simulink model "SimpleEKF_2007a"  (Simulink 6.6)
settings: Solver=FixedStepDiscrete  StartTime=0.0  StopTime=300  FixedStep=0.01  RelTol=1e-3
values from neighbouring files (symbols this model uses):
  initP = diag([ 1 1 1 1e5 1e5 1 1e5 1e5 1e5 ])    [SimpleEKF_init.m.m]
undefined symbols (not defined in the file or in its folder): DiscIntNeverNeededParam, gcbh, hwbcalib_subsystem
libraries: simulink x8, dspmtrx3 x5, dspinverses x1
(part 4 of 9)

== system SimpleEKF_2007a/INS/Coriolis correction/skewSymmetric1 ==
  skewLibIn : Inport  OutDataType=fixdt(1,16,0)  OutScaling=[]
  column1 : Selector  Tag=MBDLibrary v2007b.1  IndexOptions=Index vector (dialog)  Indices=[7 3 5]  OutputSizes=1  InputPortWidth=7  mask(Mux Selector (MBDLibrary)){InputPortWidth_mbdlib=7, Indices_mbdlib=[7 3 5]}
      mask prompts: InputPortWidth_mbdlib "Input Port Width"; Indices_mbdlib "Output Indices"
      mask help: Changes the order of the inputs.
      settings: OpenFcn=|
      | if exist('mbdlib_dialog')
      |    mbdlib_dialog(gcb,'open')
      | else
      |    open_system(gcb, 'mask')
      | end
      settings: CloseFcn=|
      | if exist('mbdlib_selector')
      |    mbdlib_selector(gcb)
      | end
      mask Help: The SELECTOR block is a MULTIPLEXED SELECTOR block, used to change the input/output order of a multiplexed data stream.
      mask Display:
      | port_label('input', 1,'[7]')
      | text(1.0,0.83333,'7', 'horizontalAlignment', 'right')
      | text(1.0,0.5,'3', 'horizontalAlignment', 'right')
      | text(1.0,0.16667,'5', 'horizontalAlignment', 'right')
  column2 : Selector  Tag=MBDLibrary v2007b.1  IndexOptions=Index vector (dialog)  Indices=[6 7 1]  OutputSizes=1  InputPortWidth=7  mask(Mux Selector (MBDLibrary)){InputPortWidth_mbdlib=7, Indices_mbdlib=[6 7 1]}
      mask prompts: InputPortWidth_mbdlib "Input Port Width"; Indices_mbdlib "Output Indices"
      mask help: Changes the order of the inputs.
      settings: OpenFcn=|
      | if exist('mbdlib_dialog')
      |    mbdlib_dialog(gcb,'open')
      | else
      |    open_system(gcb, 'mask')
      | end
      settings: CloseFcn=|
      | if exist('mbdlib_selector')
      |    mbdlib_selector(gcb)
      | end
      mask Help: The SELECTOR block is a MULTIPLEXED SELECTOR block, used to change the input/output order of a multiplexed data stream.
      mask Display:
      | port_label('input', 1,'[7]')
      | text(1.0,0.83333,'6', 'horizontalAlignment', 'right')
      | text(1.0,0.5,'7', 'horizontalAlignment', 'right')
      | text(1.0,0.16667,'1', 'horizontalAlignment', 'right')
  column3 : Selector  Tag=MBDLibrary v2007b.1  IndexOptions=Index vector (dialog)  Indices=[2 4 7]  OutputSizes=1  InputPortWidth=7  mask(Mux Selector (MBDLibrary)){InputPortWidth_mbdlib=7, Indices_mbdlib=[2 4 7]}
      mask prompts: InputPortWidth_mbdlib "Input Port Width"; Indices_mbdlib "Output Indices"
      mask help: Changes the order of the inputs.
      settings: OpenFcn=|
      | if exist('mbdlib_dialog')
      |    mbdlib_dialog(gcb,'open')
      | else
      |    open_system(gcb, 'mask')
      | end
      settings: CloseFcn=|
      | if exist('mbdlib_selector')
      |    mbdlib_selector(gcb)
      | end
      mask Help: The SELECTOR block is a MULTIPLEXED SELECTOR block, used to change the input/output order of a multiplexed data stream.
      mask Display:
      | port_label('input', 1,'[7]')
      | text(1.0,0.83333,'2', 'horizontalAlignment', 'right')
      | text(1.0,0.5,'4', 'horizontalAlignment', 'right')
      | text(1.0,0.16667,'7', 'horizontalAlignment', 'right')
  matrixConcat : Concatenate  Tag=MBDLibrary v2007b.1  NumInputs=3  Mode=Multidimensional array  ConcatenateDimension=2  mask(Matrix Concat (MBDLibrary)){concatDim=Horizontal, numInputs_mbdlib=3}
      mask prompts: concatDim "Type of Concatenate"; numInputs_mbdlib "Number of Inputs"
      mask help: Concatenate input signals of the same data type to create a contiguous output signal.
      settings: OpenFcn=|
      | if exist('mbdlib_dialog')
      |    mbdlib_dialog(gcb,'open')
      | else
      |    open_system(gcb, 'mask')
      | end
      settings: CloseFcn=|
      | if exist('mbdlib_matrixConcatenate')
      |    mbdlib_matrixConcatenate(gcb, 'mask')
      | end
      mask Help:
      | The MATRIX CONCAT block concatenates input signals from the dame data type and creates a contigouos output matrix.
      | In vector mode, all input signals must be either vectors or one-row [1xM] matrices or one-column [Mx1] matrices or a combination of vectors and either one-row matrices or one-column matrices. The output is a vector if all inputs are vectors. The output is a one-row or one-column matrix if any of the inputs are one-row or one-column matrices respectively.
      | 
      | Matrix mode treats vector inputs as one-column matrices. The output is always a matrix.
      mask StyleString: popup(Vertical|Horizontal),edit
      mask Display:
      | plot([0.1 0.3 0.3 0.1 0.1], [0.1 0.1 0.9 0.9 0.1])
      | plot([0.4 0.6 0.6 0.4 0.4], [0.1 0.1 0.9 0.9 0.1])
      | plot([0.7 0.9 0.9 0.7 0.7], [0.1 0.1 0.9 0.9 0.1])
  mux : Mux  Tag=MBDLibrary v2007b.1  Inputs=3  mask(Mux (MBDLibrary)){Inputs_mbdlib=3}
      mask prompts: Inputs_mbdlib "Number of Inputs"
      mask help: Converts multipule inputs to a vector.
      settings: OpenFcn=|
      | if exist('mbdlib_dialog')
      |    mbdlib_dialog(gcb,'open')
      | else
      |    open_system(gcb, 'mask')
      | end
      mask Help: The MUX block provides a vector output to the model for separate inputs.  The output order will correspond to the input order (from the first input at the top of the block to the last input at the bottom of the block).
  negative : Gain  Tag=MBDLibrary v2007b.1  Gain=-1  ParameterDataType=fixdt(1,16,0)  ParameterScaling=[]  OutDataType=fixdt(1,16,0)  OutScaling=[]  RndMeth=Zero  mask(Gain (MBDLibrary)){gain_mbdlib=-1}
      mask prompts: gain_mbdlib "Gain"
      mask help: Multiplies the input by the gain.
      settings: OpenFcn=|
      | if exist('mbdlib_dialog')
      |    mbdlib_dialog(gcb,'open')
      | else
      |    open_system(gcb, 'mask')
      | end
      mask Help: The GAIN block multiplies the input by the gain value.  This block may accept any data types other than boolean.  The user must take care to not use a non-integer gain for int32/uint32 inputs.
      mask Display: disp([get_param(gcb, 'Gain') 'x'])
  zero : Constant  Tag=MBDLibrary v2007b.1  Value=0  VectorParams1D=off  OutDataType=fixdt(1,16,0)  OutScaling=[]  mask(Constant (MBDLibrary)){Value_mbdlib=0, OutDataTypeMode_mbdlib=double}
      mask prompts: Value_mbdlib "Constant"; OutDataTypeMode_mbdlib "Data Type"
      mask help: Outputs a constant value
      settings: AttributesFormatString={%<OutDataTypeMode>}
      settings: OpenFcn=|
      | if exist('mbdlib_dialog')
      |    mbdlib_dialog(gcb,'open')
      | else
      |    open_system(gcb, 'mask')
      | end
      settings: CloseFcn=|
      | if exist('mbdlib_dialog')
      |    mbdlib_constant(gcb)
      | end
      mask Help: The CONSTANT block outputs a constant value to the system.
      mask StyleString: edit,popup(double|single|boolean|int32|uint32)
  skewLibOut : Outport  OutDataType=fixdt(1,16,0)  OutScaling=[]
  wires:
  zero/1 -> mux/3
  negative/1 -> mux/2
  column3/1 -> matrixConcat/3
  column2/1 -> matrixConcat/2
  column1/1 -> matrixConcat/1
  matrixConcat/1 -> skewLibOut/1
  mux/1 -> column1/1, column3/1, column2/1
  skewLibIn/1 -> mux/1, negative/1

== system SimpleEKF_2007a/INS/Gravity/square ==
  squareLibIn : Inport  DataType=double  OutDataType=fixdt(1,16,0)  OutScaling=[]
  Product : Product  OutDataType=fixdt(1,16,0)  OutScaling=[]  RndMeth=Zero
  squareLibOut : Outport  OutDataType=fixdt(1,16,0)  OutScaling=[]  InitialOutput=0
  wires:
  squareLibIn/1 -> Product/2, Product/1
  Product/1 -> squareLibOut/1

== system SimpleEKF_2007a/INS/Gravity/square1 ==
  squareLibIn : Inport  DataType=double  OutDataType=fixdt(1,16,0)  OutScaling=[]
  Product : Product  OutDataType=fixdt(1,16,0)  OutScaling=[]  RndMeth=Zero
  squareLibOut : Outport  OutDataType=fixdt(1,16,0)  OutScaling=[]  InitialOutput=0
  wires:
  squareLibIn/1 -> Product/2, Product/1
  Product/1 -> squareLibOut/1

== system SimpleEKF_2007a/INS/Gravity/square2 ==
  squareLibIn : Inport  DataType=double  OutDataType=fixdt(1,16,0)  OutScaling=[]
  Product : Product  OutDataType=fixdt(1,16,0)  OutScaling=[]  RndMeth=Zero
  squareLibOut : Outport  OutDataType=fixdt(1,16,0)  OutScaling=[]  InitialOutput=0
  wires:
  squareLibIn/1 -> Product/2, Product/1
  Product/1 -> squareLibOut/1

== system SimpleEKF_2007a/INS/Gravity/square3 ==
  squareLibIn : Inport  DataType=double  OutDataType=fixdt(1,16,0)  OutScaling=[]
  Product : Product  OutDataType=fixdt(1,16,0)  OutScaling=[]  RndMeth=Zero
  squareLibOut : Outport  OutDataType=fixdt(1,16,0)  OutScaling=[]  InitialOutput=0
  wires:
  squareLibIn/1 -> Product/2, Product/1
  Product/1 -> squareLibOut/1

== system SimpleEKF_2007a/INS/Gravity/square4 ==
  squareLibIn : Inport  DataType=double  OutDataType=fixdt(1,16,0)  OutScaling=[]
  Product : Product  OutDataType=fixdt(1,16,0)  OutScaling=[]  RndMeth=Zero
  squareLibOut : Outport  OutDataType=fixdt(1,16,0)  OutScaling=[]  InitialOutput=0
  wires:
  squareLibIn/1 -> Product/2, Product/1
  Product/1 -> squareLibOut/1

== system SimpleEKF_2007a/INS/Velocity update/acc from BODY to NAV ==
  acc_Body : Inport  PortDimensions=3  SampleTime=0.01  OutDataType=fixdt(1,16,0)  OutScaling=[]
  dcmBodyToNav : Inport  Port=2  PortDimensions=[3,3]  SampleTime=0.01  OutDataType=fixdt(1,16,0)  OutScaling=[]
  Matrix Multiply : Product  Multiplication=Matrix(*)  OutDataType=fixdt(1,16,0)  OutScaling=[]
  acc_Nav : Outport  PortDimensions=3  SampleTime=0.01  OutDataType=fixdt(1,16,0)  OutScaling=[]
  wires:
  dcmBodyToNav/1 -> Matrix Multiply/1
  Matrix Multiply/1 -> acc_Nav/1
  acc_Body/1 -> Matrix Multiply/2

== system SimpleEKF_2007a/INS/Velocity update/acc(k-1) from BODY to NAV ==
  acc_Body : Inport  OutDataType=fixdt(1,16,0)  OutScaling=[]
  dcmBodyToNav : Inport  Port=2  OutDataType=fixdt(1,16,0)  OutScaling=[]
  Matrix Multiply : Product  Multiplication=Matrix(*)  OutDataType=fixdt(1,16,0)  OutScaling=[]
  acc_Nav(k-1) : Outport  OutDataType=fixdt(1,16,0)  OutScaling=[]
  wires:
  dcmBodyToNav/1 -> Matrix Multiply/1
  Matrix Multiply/1 -> acc_Nav(k-1)/1
  acc_Body/1 -> Matrix Multiply/2

== system SimpleEKF_2007a/Trajectory  Generator/Signals Conversions dtgen/Axes and WA correction ==
  note: Axes and WA correction
  note: NED (WA) -> NED
  note: ENU frame (WA) -> NED frame (WA)
  note: ENU frame (WA)
  velWan : Inport  OutDataType=fixdt(1,16,0)  OutScaling=[]
  alpha : Inport  Port=2  OutDataType=fixdt(1,16,0)  OutScaling=[]
  -vnz : Gain  Gain=-1  ParameterDataType=fixdt(1,16,0)  ParameterScaling=[]  OutDataType=fixdt(1,16,0)  OutScaling=[]
  Bus Creator : BusCreator  Inputs=3
  Bus Creator1 : BusCreator  Inputs=3
  Bus Selector : BusSelector  OutputSignals=x,y,z
  Bus Selector1 : BusSelector  OutputSignals=y,x,z
  Mux : Mux
  c1 : Fcn  Expr=u[1]*sin(u[4]) + u[2]*cos(u[4])
  c2 : Fcn  Expr=u[3]
  c6 : Fcn  Expr=u[1]*cos(u[4]) - u[2]*sin(u[4])
  velNav : Outport  OutDataType=fixdt(1,16,0)  OutScaling=[]
  wires:
  alpha/1 -> Mux/4  "wanAng"
  -vnz/1 -> Mux/3  "vnz [m/s]"
  Bus Selector1/3 -> -vnz/1  "<z>"
  Bus Selector/3 -> Bus Creator/3  "<z>"
  c2/1 -> Bus Creator1/3  "down"
  Bus Creator1/1 -> velNav/1  "velNavTrue"
  c1/1 -> Bus Creator1/2  "east"
  c6/1 -> Bus Creator1/1  "north"
  Mux/1 -> c1/1, c2/1, c6/1
  Bus Selector1/2 -> Mux/2  "<x>"
  Bus Selector1/1 -> Mux/1  "<y>"
  Bus Creator/1 -> Bus Selector1/1
  Bus Selector/2 -> Bus Creator/2  "<y>"
  Bus Selector/1 -> Bus Creator/1  "<x>"
  velWan/1 -> Bus Selector/1

== system SimpleEKF_2007a/Trajectory  Generator/Signals Conversions dtgen/Subsystem1 ==
  note: Equation for Transforming Geodetic Coordinate
      | to Rectangular (ECEF) coordinates:
      | (NIMA TR8350.2 Third Edition, 3 January 2000)
      |
      | Equation 4-14:
      | x_{ECEF} = (N + h)cos(\lambda)cos(\Lambda)
      | y_{ECEF} = (N + h)cos(\lambda)sin(\Lambda)
      | z_{ECEF} = ((b/a)^2N + h)sin(\lambda)
      |
      | Equation 4-15:
      | N = a / (1-e^2sin^2(\lambda))^{1/2}
      |
      | Where:
      | (\lambda, \Lambda, h) = geodetic coordinates (in meters & rad)
      | b/a = earth axis ratio
      | a = earth semi-major axis (in m)
      | e = earth first eccentricity
  geoToECEFLibInLon : Inport  OutDataType=fixdt(1,16,0)  OutScaling=[]
  geoToECEFLibInLat : Inport  Port=2  OutDataType=fixdt(1,16,0)  OutScaling=[]
  geoToECEFLibInAlt : Inport  Port=3  OutDataType=fixdt(1,16,0)  OutScaling=[]
  Math Function : Math  Operator=reciprocal  OutDataType=fixdt(1,16,0)  OutScaling=[]  SaturateOnIntegerOverflow=on
  Sqrt : Math  Operator=sqrt  OutDataType=fixdt(1,16,0)  OutScaling=[]  SaturateOnIntegerOverflow=on
  Trigonometric Function : Trigonometry  Operator=cos
  Trigonometric Function1 : Trigonometry  Operator=cos
  Trigonometric Function2 : Trigonometry
  Trigonometric Function3 : Trigonometry
  axisRatio : Gain  Tag=MBDLibrary v2007b.1  Gain=.996647189335^2  ParameterDataType=fixdt(1,16,0)  ParameterScaling=[]  OutDataType=fixdt(1,16,0)  OutScaling=[]  RndMeth=Zero  mask(Gain (MBDLibrary)){gain_mbdlib=.996647189335^2}
      mask prompts: gain_mbdlib "Gain"
      mask help: Multiplies the input by the gain.
      settings: OpenFcn=|
      | if exist('mbdlib_dialog')
      |    mbdlib_dialog(gcb,'open')
      | else
      |    open_system(gcb, 'mask')
      | end
      mask Help: The GAIN block multiplies the input by the gain value.  This block may accept any data types other than boolean.  The user must take care to not use a non-integer gain for int32/uint32 inputs.
      mask Display: disp([get_param(gcb, 'Gain') 'x'])
  bias : Bias  Tag=MBDLibrary v2007b.1  Bias=1  mask(Bias (MBDLibrary)){Bias_mbdlib=1}
      mask prompts: Bias_mbdlib "Bias"
      mask help: Add bias to input.
      settings: OpenFcn=|
      | if exist('mbdlib_dialog')
      |    mbdlib_dialog(gcb,'open')
      | else
      |    open_system(gcb, 'mask')
      | end
      settings: CloseFcn=|
      | if exist('mbdlib_bias')
      |    mbdlib_bias(gcb)
      | end
      mask Help: The BIAS block outputs the summation of an input with a specified constant.
      mask Display: disp(['x+1'])
  eqPlane : Product  Tag=MBDLibrary v2007b.1  OutDataType=fixdt(1,16,0)  OutScaling=[]  RndMeth=Zero  InputSameDT=on  mask(Product (MBDLibrary)){Inputs_mbdlib=2}
      mask prompts: Inputs_mbdlib "Number of Inputs"
      mask help: Multiplies inputs.
      settings: OpenFcn=|
      | if exist('mbdlib_dialog')
      |    mbdlib_dialog(gcb,'open')
      | else
      |    open_system(gcb, 'mask')
      | end
      mask Help: The PRODUCT block is used to multiply inputs.
  firstEccentricitySquared : Gain  Tag=MBDLibrary v2007b.1  Gain=-6.69437999014e-3  ParameterDataType=fixdt(1,16,0)  ParameterScaling=[]  OutDataType=fixdt(1,16,0)  OutScaling=[]  RndMeth=Zero  mask(Gain (MBDLibrary)){gain_mbdlib=-6.69437999014e-3}
      mask prompts: gain_mbdlib "Gain"
      mask help: Multiplies the input by the gain.
      settings: OpenFcn=|
      | if exist('mbdlib_dialog')
      |    mbdlib_dialog(gcb,'open')
      | else
      |    open_system(gcb, 'mask')
      | end
      mask Help: The GAIN block multiplies the input by the gain value.  This block may accept any data types other than boolean.  The user must take care to not use a non-integer gain for int32/uint32 inputs.
      mask Display: disp([get_param(gcb, 'Gain') 'x'])
  gain : Gain  Tag=MBDLibrary v2007b.1  Gain=6378137.0  ParameterDataType=fixdt(1,16,0)  ParameterScaling=[]  OutDataType=fixdt(1,16,0)  OutScaling=[]  RndMeth=Zero  mask(Gain (MBDLibrary)){gain_mbdlib=6378137.0}
      mask prompts: gain_mbdlib "Gain"
      mask help: Multiplies the input by the gain.
      settings: OpenFcn=|
      | if exist('mbdlib_dialog')
      |    mbdlib_dialog(gcb,'open')
      | else
      |    open_system(gcb, 'mask')
      | end
      mask Help: The GAIN block multiplies the input by the gain value.  This block may accept any data types other than boolean.  The user must take care to not use a non-integer gain for int32/uint32 inputs.
      mask Display: disp([get_param(gcb, 'Gain') 'x'])
  radius : Sum  Tag=MBDLibrary v2007b.1  OutDataType=fixdt(1,16,0)  OutScaling=[]  RndMeth=Zero  InputSameDT=on  mask(Sum (MBDLibrary)){inputs_mbdlib=++}
      mask prompts: inputs_mbdlib "List of signs"
      mask help: Adds values together.
      settings: OpenFcn=|
      | if exist('mbdlib_dialog')
      |    mbdlib_dialog(gcb,'open')
      | else
      |    open_system(gcb, 'mask')
      | end
      mask Help:
      | The SUM block is used to add or subtract  inputs.
      | The inputs may be specified as:
      |   (a) + or - for each port (i.e. ++-+)
      |   (b) An integer to indicate the number of ports to add
      | Note that the number of ports input to this block must be between 1 and 25.
      | When only 1 inport is selected, the block computes the summation of vector input elements and outputs a scalar.
  radius1 : Sum  Tag=MBDLibrary v2007b.1  OutDataType=fixdt(1,16,0)  OutScaling=[]  RndMeth=Zero  InputSameDT=on  mask(Sum (MBDLibrary)){inputs_mbdlib=++}
      mask prompts: inputs_mbdlib "List of signs"
      mask help: Adds values together.
      settings: OpenFcn=|
      | if exist('mbdlib_dialog')
      |    mbdlib_dialog(gcb,'open')
      | else
      |    open_system(gcb, 'mask')
      | end
      mask Help:
      | The SUM block is used to add or subtract  inputs.
      | The inputs may be specified as:
      |   (a) + or - for each port (i.e. ++-+)
      |   (b) An integer to indicate the number of ports to add
      | Note that the number of ports input to this block must be between 1 and 25.
      | When only 1 inport is selected, the block computes the summation of vector input elements and outputs a scalar.
  square : Subsystem  Tag=MBDLibrary v2007b.1
      settings: OpenFcn=|
      | if exist('mbdlib_dialog')
      |    mbdlib_dialog(gcb,'open')
      | else
      |    open_system(gcb, 'mask')
      | end
      mask Type: Square (MBDLibrary)
      mask Description: Squares the input.
      mask Help: The SQAURE block outputs the square of the input value.
      mask Display: disp('x^2', 'texmode', 'on')
  xECEF : Product  Tag=MBDLibrary v2007b.1  OutDataType=fixdt(1,16,0)  OutScaling=[]  RndMeth=Zero  InputSameDT=on  mask(Product (MBDLibrary)){Inputs_mbdlib=2}
      mask prompts: Inputs_mbdlib "Number of Inputs"
      mask help: Multiplies inputs.
      settings: OpenFcn=|
      | if exist('mbdlib_dialog')
      |    mbdlib_dialog(gcb,'open')
      | else
      |    open_system(gcb, 'mask')
      | end
      mask Help: The PRODUCT block is used to multiply inputs.
  yECEF : Product  Tag=MBDLibrary v2007b.1  OutDataType=fixdt(1,16,0)  OutScaling=[]  RndMeth=Zero  InputSameDT=on  mask(Product (MBDLibrary)){Inputs_mbdlib=2}
      mask prompts: Inputs_mbdlib "Number of Inputs"
      mask help: Multiplies inputs.
      settings: OpenFcn=|
      | if exist('mbdlib_dialog')
      |    mbdlib_dialog(gcb,'open')
      | else
      |    open_system(gcb, 'mask')
      | end
      mask Help: The PRODUCT block is used to multiply inputs.
  zECEF : Product  Tag=MBDLibrary v2007b.1  OutDataType=fixdt(1,16,0)  OutScaling=[]  RndMeth=Zero  InputSameDT=on  mask(Product (MBDLibrary)){Inputs_mbdlib=2}
      mask prompts: Inputs_mbdlib "Number of Inputs"
      mask help: Multiplies inputs.
      settings: OpenFcn=|
      | if exist('mbdlib_dialog')
      |    mbdlib_dialog(gcb,'open')
      | else
      |    open_system(gcb, 'mask')
      | end
      mask Help: The PRODUCT block is used to multiply inputs.
  geoToECEFLibOutX : Outport  OutDataType=fixdt(1,16,0)  OutScaling=[]
  geoToECEFLibOutY : Outport  Port=2  OutDataType=fixdt(1,16,0)  OutScaling=[]
  geoToECEFLibOutZ : Outport  Port=3  OutDataType=fixdt(1,16,0)  OutScaling=[]
  wires:
  Trigonometric Function3/1 -> zECEF/2, square/1(squareLibIn)
  zECEF/1 -> geoToECEFLibOutZ/1
  yECEF/1 -> geoToECEFLibOutY/1
  xECEF/1 -> geoToECEFLibOutX/1
  radius1/1 -> zECEF/1
  eqPlane/1 -> yECEF/2, xECEF/1
  Trigonometric Function2/1 -> yECEF/1
  geoToECEFLibInLon/1 -> Trigonometric Function1/1, Trigonometric Function2/1
  axisRatio/1 -> radius1/2
  geoToECEFLibInAlt/1 -> radius1/1, radius/2
  gain/1 -> axisRatio/1, radius/1
  Trigonometric Function/1 -> eqPlane/1
  Trigonometric Function1/1 -> xECEF/2
  radius/1 -> eqPlane/2
  bias/1 -> Sqrt/1
  firstEccentricitySquared/1 -> bias/1
  square/1(squareLibOut) -> firstEccentricitySquared/1
  geoToECEFLibInLat/1 -> Trigonometric Function/1, Trigonometric Function3/1
  Sqrt/1 -> Math Function/1
  Math Function/1 -> gain/1

== system SimpleEKF_2007a/EKF/MeasureVector/GPS/Subsystem1 ==
  note: Equation for Transforming Geodetic Coordinate
      | to Rectangular (ECEF) coordinates:
      | (NIMA TR8350.2 Third Edition, 3 January 2000)
      |
      | Equation 4-14:
      | x_{ECEF} = (N + h)cos(\lambda)cos(\Lambda)
      | y_{ECEF} = (N + h)cos(\lambda)sin(\Lambda)
      | z_{ECEF} = ((b/a)^2N + h)sin(\lambda)
      |
      | Equation 4-15:
      | N = a / (1-e^2sin^2(\lambda))^{1/2}
      |
      | Where:
      | (\lambda, \Lambda, h) = geodetic coordinates (in meters & rad)
      | b/a = earth axis ratio
      | a = earth semi-major axis (in m)
      | e = earth first eccentricity
  geoToECEFLibInLon : Inport  OutDataType=fixdt(1,16,0)  OutScaling=[]
  geoToECEFLibInLat : Inport  Port=2  OutDataType=fixdt(1,16,0)  OutScaling=[]
  geoToECEFLibInAlt : Inport  Port=3  OutDataType=fixdt(1,16,0)  OutScaling=[]
  Math Function : Math  Operator=reciprocal  OutDataType=fixdt(1,16,0)  OutScaling=[]  SaturateOnIntegerOverflow=on
  Sqrt : Math  Operator=sqrt  OutDataType=fixdt(1,16,0)  OutScaling=[]  SaturateOnIntegerOverflow=on
  Trigonometric Function : Trigonometry  Operator=cos
  Trigonometric Function1 : Trigonometry  Operator=cos
  Trigonometric Function2 : Trigonometry
  Trigonometric Function3 : Trigonometry
  axisRatio : Gain  Tag=MBDLibrary v2007b.1  Gain=.996647189335^2  ParameterDataType=fixdt(1,16,0)  ParameterScaling=[]  OutDataType=fixdt(1,16,0)  OutScaling=[]  RndMeth=Zero  mask(Gain (MBDLibrary)){gain_mbdlib=.996647189335^2}
      mask prompts: gain_mbdlib "Gain"
      mask help: Multiplies the input by the gain.
      settings: OpenFcn=|
      | if exist('mbdlib_dialog')
      |    mbdlib_dialog(gcb,'open')
      | else
      |    open_system(gcb, 'mask')
      | end
      mask Help: The GAIN block multiplies the input by the gain value.  This block may accept any data types other than boolean.  The user must take care to not use a non-integer gain for int32/uint32 inputs.
      mask Display: disp([get_param(gcb, 'Gain') 'x'])
  bias : Bias  Tag=MBDLibrary v2007b.1  Bias=1  mask(Bias (MBDLibrary)){Bias_mbdlib=1}
      mask prompts: Bias_mbdlib "Bias"
      mask help: Add bias to input.
      settings: OpenFcn=|
      | if exist('mbdlib_dialog')
      |    mbdlib_dialog(gcb,'open')
      | else
      |    open_system(gcb, 'mask')
      | end
      settings: CloseFcn=|
      | if exist('mbdlib_bias')
      |    mbdlib_bias(gcb)
      | end
      mask Help: The BIAS block outputs the summation of an input with a specified constant.
      mask Display: disp(['x+1'])
  eqPlane : Product  Tag=MBDLibrary v2007b.1  OutDataType=fixdt(1,16,0)  OutScaling=[]  RndMeth=Zero  InputSameDT=on  mask(Product (MBDLibrary)){Inputs_mbdlib=2}
      mask prompts: Inputs_mbdlib "Number of Inputs"
      mask help: Multiplies inputs.
      settings: OpenFcn=|
      | if exist('mbdlib_dialog')
      |    mbdlib_dialog(gcb,'open')
      | else
      |    open_system(gcb, 'mask')
      | end
      mask Help: The PRODUCT block is used to multiply inputs.
  firstEccentricitySquared : Gain  Tag=MBDLibrary v2007b.1  Gain=-6.69437999014e-3  ParameterDataType=fixdt(1,16,0)  ParameterScaling=[]  OutDataType=fixdt(1,16,0)  OutScaling=[]  RndMeth=Zero  mask(Gain (MBDLibrary)){gain_mbdlib=-6.69437999014e-3}
      mask prompts: gain_mbdlib "Gain"
      mask help: Multiplies the input by the gain.
      settings: OpenFcn=|
      | if exist('mbdlib_dialog')
      |    mbdlib_dialog(gcb,'open')
      | else
      |    open_system(gcb, 'mask')
      | end
      mask Help: The GAIN block multiplies the input by the gain value.  This block may accept any data types other than boolean.  The user must take care to not use a non-integer gain for int32/uint32 inputs.
      mask Display: disp([get_param(gcb, 'Gain') 'x'])
  gain : Gain  Tag=MBDLibrary v2007b.1  Gain=6378137.0  ParameterDataType=fixdt(1,16,0)  ParameterScaling=[]  OutDataType=fixdt(1,16,0)  OutScaling=[]  RndMeth=Zero  mask(Gain (MBDLibrary)){gain_mbdlib=6378137.0}
      mask prompts: gain_mbdlib "Gain"
      mask help: Multiplies the input by the gain.
      settings: OpenFcn=|
      | if exist('mbdlib_dialog')
      |    mbdlib_dialog(gcb,'open')
      | else
      |    open_system(gcb, 'mask')
      | end
      mask Help: The GAIN block multiplies the input by the gain value.  This block may accept any data types other than boolean.  The user must take care to not use a non-integer gain for int32/uint32 inputs.
      mask Display: disp([get_param(gcb, 'Gain') 'x'])
  radius : Sum  Tag=MBDLibrary v2007b.1  OutDataType=fixdt(1,16,0)  OutScaling=[]  RndMeth=Zero  InputSameDT=on  mask(Sum (MBDLibrary)){inputs_mbdlib=++}
      mask prompts: inputs_mbdlib "List of signs"
      mask help: Adds values together.
      settings: OpenFcn=|
      | if exist('mbdlib_dialog')
      |    mbdlib_dialog(gcb,'open')
      | else
      |    open_system(gcb, 'mask')
      | end
      mask Help:
      | The SUM block is used to add or subtract  inputs.
      | The inputs may be specified as:
      |   (a) + or - for each port (i.e. ++-+)
      |   (b) An integer to indicate the number of ports to add
      | Note that the number of ports input to this block must be between 1 and 25.
      | When only 1 inport is selected, the block computes the summation of vector input elements and outputs a scalar.
  radius1 : Sum  Tag=MBDLibrary v2007b.1  OutDataType=fixdt(1,16,0)  OutScaling=[]  RndMeth=Zero  InputSameDT=on  mask(Sum (MBDLibrary)){inputs_mbdlib=++}
      mask prompts: inputs_mbdlib "List of signs"
      mask help: Adds values together.
      settings: OpenFcn=|
      | if exist('mbdlib_dialog')
      |    mbdlib_dialog(gcb,'open')
      | else
      |    open_system(gcb, 'mask')
      | end
      mask Help:
      | The SUM block is used to add or subtract  inputs.
      | The inputs may be specified as:
      |   (a) + or - for each port (i.e. ++-+)
      |   (b) An integer to indicate the number of ports to add
      | Note that the number of ports input to this block must be between 1 and 25.
      | When only 1 inport is selected, the block computes the summation of vector input elements and outputs a scalar.
  square : Subsystem  Tag=MBDLibrary v2007b.1
      settings: OpenFcn=|
      | if exist('mbdlib_dialog')
      |    mbdlib_dialog(gcb,'open')
      | else
      |    open_system(gcb, 'mask')
      | end
      mask Type: Square (MBDLibrary)
      mask Description: Squares the input.
      mask Help: The SQAURE block outputs the square of the input value.
      mask Display: disp('x^2', 'texmode', 'on')
  xECEF : Product  Tag=MBDLibrary v2007b.1  OutDataType=fixdt(1,16,0)  OutScaling=[]  RndMeth=Zero  InputSameDT=on  mask(Product (MBDLibrary)){Inputs_mbdlib=2}
      mask prompts: Inputs_mbdlib "Number of Inputs"
      mask help: Multiplies inputs.
      settings: OpenFcn=|
      | if exist('mbdlib_dialog')
      |    mbdlib_dialog(gcb,'open')
      | else
      |    open_system(gcb, 'mask')
      | end
      mask Help: The PRODUCT block is used to multiply inputs.
  yECEF : Product  Tag=MBDLibrary v2007b.1  OutDataType=fixdt(1,16,0)  OutScaling=[]  RndMeth=Zero  InputSameDT=on  mask(Product (MBDLibrary)){Inputs_mbdlib=2}
      mask prompts: Inputs_mbdlib "Number of Inputs"
      mask help: Multiplies inputs.
      settings: OpenFcn=|
      | if exist('mbdlib_dialog')
      |    mbdlib_dialog(gcb,'open')
      | else
      |    open_system(gcb, 'mask')
      | end
      mask Help: The PRODUCT block is used to multiply inputs.
  zECEF : Product  Tag=MBDLibrary v2007b.1  OutDataType=fixdt(1,16,0)  OutScaling=[]  RndMeth=Zero  InputSameDT=on  mask(Product (MBDLibrary)){Inputs_mbdlib=2}
      mask prompts: Inputs_mbdlib "Number of Inputs"
      mask help: Multiplies inputs.
      settings: OpenFcn=|
      | if exist('mbdlib_dialog')
      |    mbdlib_dialog(gcb,'open')
      | else
      |    open_system(gcb, 'mask')
      | end
      mask Help: The PRODUCT block is used to multiply inputs.
  geoToECEFLibOutX : Outport  OutDataType=fixdt(1,16,0)  OutScaling=[]
  geoToECEFLibOutY : Outport  Port=2  OutDataType=fixdt(1,16,0)  OutScaling=[]
  geoToECEFLibOutZ : Outport  Port=3  OutDataType=fixdt(1,16,0)  OutScaling=[]
  wires:
  Trigonometric Function3/1 -> zECEF/2, square/1(squareLibIn)
  zECEF/1 -> geoToECEFLibOutZ/1
  yECEF/1 -> geoToECEFLibOutY/1
  xECEF/1 -> geoToECEFLibOutX/1
  radius1/1 -> zECEF/1
  eqPlane/1 -> yECEF/2, xECEF/1
  Trigonometric Function2/1 -> yECEF/1
  geoToECEFLibInLon/1 -> Trigonometric Function1/1, Trigonometric Function2/1
  axisRatio/1 -> radius1/2
  geoToECEFLibInAlt/1 -> radius1/1, radius/2
  gain/1 -> axisRatio/1, radius/1
  Trigonometric Function/1 -> eqPlane/1
  Trigonometric Function1/1 -> xECEF/2
  radius/1 -> eqPlane/2
  bias/1 -> Sqrt/1
  firstEccentricitySquared/1 -> bias/1
  square/1(squareLibOut) -> firstEccentricitySquared/1
  geoToECEFLibInLat/1 -> Trigonometric Function/1, Trigonometric Function3/1
  Sqrt/1 -> Math Function/1
  Math Function/1 -> gain/1

== system SimpleEKF_2007a/EKF/MeasureVector/GPS/Subsystem2 ==
  note: Equation for Transforming Geodetic Coordinate
      | to Rectangular (ECEF) coordinates:
      | (NIMA TR8350.2 Third Edition, 3 January 2000)
      |
      | Equation 4-14:
      | x_{ECEF} = (N + h)cos(\lambda)cos(\Lambda)
      | y_{ECEF} = (N + h)cos(\lambda)sin(\Lambda)
      | z_{ECEF} = ((b/a)^2N + h)sin(\lambda)
      |
      | Equation 4-15:
      | N = a / (1-e^2sin^2(\lambda))^{1/2}
      |
      | Where:
      | (\lambda, \Lambda, h) = geodetic coordinates (in meters & rad)
      | b/a = earth axis ratio
      | a = earth semi-major axis (in m)
      | e = earth first eccentricity
  geoToECEFLibInLon : Inport  OutDataType=fixdt(1,16,0)  OutScaling=[]
  geoToECEFLibInLat : Inport  Port=2  OutDataType=fixdt(1,16,0)  OutScaling=[]
  geoToECEFLibInAlt : Inport  Port=3  OutDataType=fixdt(1,16,0)  OutScaling=[]
  Math Function : Math  Operator=reciprocal  OutDataType=fixdt(1,16,0)  OutScaling=[]  SaturateOnIntegerOverflow=on
  Sqrt : Math  Operator=sqrt  OutDataType=fixdt(1,16,0)  OutScaling=[]  SaturateOnIntegerOverflow=on
  Trigonometric Function : Trigonometry  Operator=cos
  Trigonometric Function1 : Trigonometry  Operator=cos
  Trigonometric Function2 : Trigonometry
  Trigonometric Function3 : Trigonometry
  axisRatio : Gain  Tag=MBDLibrary v2007b.1  Gain=.996647189335^2  ParameterDataType=fixdt(1,16,0)  ParameterScaling=[]  OutDataType=fixdt(1,16,0)  OutScaling=[]  RndMeth=Zero  mask(Gain (MBDLibrary)){gain_mbdlib=.996647189335^2}
      mask prompts: gain_mbdlib "Gain"
      mask help: Multiplies the input by the gain.
      settings: OpenFcn=|
      | if exist('mbdlib_dialog')
      |    mbdlib_dialog(gcb,'open')
      | else
      |    open_system(gcb, 'mask')
      | end
      mask Help: The GAIN block multiplies the input by the gain value.  This block may accept any data types other than boolean.  The user must take care to not use a non-integer gain for int32/uint32 inputs.
      mask Display: disp([get_param(gcb, 'Gain') 'x'])
  bias : Bias  Tag=MBDLibrary v2007b.1  Bias=1  mask(Bias (MBDLibrary)){Bias_mbdlib=1}
      mask prompts: Bias_mbdlib "Bias"
      mask help: Add bias to input.
      settings: OpenFcn=|
      | if exist('mbdlib_dialog')
      |    mbdlib_dialog(gcb,'open')
      | else
      |    open_system(gcb, 'mask')
      | end
      settings: CloseFcn=|
      | if exist('mbdlib_bias')
      |    mbdlib_bias(gcb)
      | end
      mask Help: The BIAS block outputs the summation of an input with a specified constant.
      mask Display: disp(['x+1'])
  eqPlane : Product  Tag=MBDLibrary v2007b.1  OutDataType=fixdt(1,16,0)  OutScaling=[]  RndMeth=Zero  InputSameDT=on  mask(Product (MBDLibrary)){Inputs_mbdlib=2}
      mask prompts: Inputs_mbdlib "Number of Inputs"
      mask help: Multiplies inputs.
      settings: OpenFcn=|
      | if exist('mbdlib_dialog')
      |    mbdlib_dialog(gcb,'open')
      | else
      |    open_system(gcb, 'mask')
      | end
      mask Help: The PRODUCT block is used to multiply inputs.
  firstEccentricitySquared : Gain  Tag=MBDLibrary v2007b.1  Gain=-6.69437999014e-3  ParameterDataType=fixdt(1,16,0)  ParameterScaling=[]  OutDataType=fixdt(1,16,0)  OutScaling=[]  RndMeth=Zero  mask(Gain (MBDLibrary)){gain_mbdlib=-6.69437999014e-3}
      mask prompts: gain_mbdlib "Gain"
      mask help: Multiplies the input by the gain.
      settings: OpenFcn=|
      | if exist('mbdlib_dialog')
      |    mbdlib_dialog(gcb,'open')
      | else
      |    open_system(gcb, 'mask')
      | end
      mask Help: The GAIN block multiplies the input by the gain value.  This block may accept any data types other than boolean.  The user must take care to not use a non-integer gain for int32/uint32 inputs.
      mask Display: disp([get_param(gcb, 'Gain') 'x'])
  gain : Gain  Tag=MBDLibrary v2007b.1  Gain=6378137.0  ParameterDataType=fixdt(1,16,0)  ParameterScaling=[]  OutDataType=fixdt(1,16,0)  OutScaling=[]  RndMeth=Zero  mask(Gain (MBDLibrary)){gain_mbdlib=6378137.0}
      mask prompts: gain_mbdlib "Gain"
      mask help: Multiplies the input by the gain.
      settings: OpenFcn=|
      | if exist('mbdlib_dialog')
      |    mbdlib_dialog(gcb,'open')
      | else
      |    open_system(gcb, 'mask')
      | end
      mask Help: The GAIN block multiplies the input by the gain value.  This block may accept any data types other than boolean.  The user must take care to not use a non-integer gain for int32/uint32 inputs.
      mask Display: disp([get_param(gcb, 'Gain') 'x'])
  radius : Sum  Tag=MBDLibrary v2007b.1  OutDataType=fixdt(1,16,0)  OutScaling=[]  RndMeth=Zero  InputSameDT=on  mask(Sum (MBDLibrary)){inputs_mbdlib=++}
      mask prompts: inputs_mbdlib "List of signs"
      mask help: Adds values together.
      settings: OpenFcn=|
      | if exist('mbdlib_dialog')
      |    mbdlib_dialog(gcb,'open')
      | else
      |    open_system(gcb, 'mask')
      | end
      mask Help:
      | The SUM block is used to add or subtract  inputs.
      | The inputs may be specified as:
      |   (a) + or - for each port (i.e. ++-+)
      |   (b) An integer to indicate the number of ports to add
      | Note that the number of ports input to this block must be between 1 and 25.
      | When only 1 inport is selected, the block computes the summation of vector input elements and outputs a scalar.
  radius1 : Sum  Tag=MBDLibrary v2007b.1  OutDataType=fixdt(1,16,0)  OutScaling=[]  RndMeth=Zero  InputSameDT=on  mask(Sum (MBDLibrary)){inputs_mbdlib=++}
      mask prompts: inputs_mbdlib "List of signs"
      mask help: Adds values together.
      settings: OpenFcn=|
      | if exist('mbdlib_dialog')
      |    mbdlib_dialog(gcb,'open')
      | else
      |    open_system(gcb, 'mask')
      | end
      mask Help:
      | The SUM block is used to add or subtract  inputs.
      | The inputs may be specified as:
      |   (a) + or - for each port (i.e. ++-+)
      |   (b) An integer to indicate the number of ports to add
      | Note that the number of ports input to this block must be between 1 and 25.
      | When only 1 inport is selected, the block computes the summation of vector input elements and outputs a scalar.
  square : Subsystem  Tag=MBDLibrary v2007b.1
      settings: OpenFcn=|
      | if exist('mbdlib_dialog')
      |    mbdlib_dialog(gcb,'open')
      | else
      |    open_system(gcb, 'mask')
      | end
      mask Type: Square (MBDLibrary)
      mask Description: Squares the input.
      mask Help: The SQAURE block outputs the square of the input value.
      mask Display: disp('x^2', 'texmode', 'on')
  xECEF : Product  Tag=MBDLibrary v2007b.1  OutDataType=fixdt(1,16,0)  OutScaling=[]  RndMeth=Zero  InputSameDT=on  mask(Product (MBDLibrary)){Inputs_mbdlib=2}
      mask prompts: Inputs_mbdlib "Number of Inputs"
      mask help: Multiplies inputs.
      settings: OpenFcn=|
      | if exist('mbdlib_dialog')
      |    mbdlib_dialog(gcb,'open')
      | else
      |    open_system(gcb, 'mask')
      | end
      mask Help: The PRODUCT block is used to multiply inputs.
  yECEF : Product  Tag=MBDLibrary v2007b.1  OutDataType=fixdt(1,16,0)  OutScaling=[]  RndMeth=Zero  InputSameDT=on  mask(Product (MBDLibrary)){Inputs_mbdlib=2}
      mask prompts: Inputs_mbdlib "Number of Inputs"
      mask help: Multiplies inputs.
      settings: OpenFcn=|
      | if exist('mbdlib_dialog')
      |    mbdlib_dialog(gcb,'open')
      | else
      |    open_system(gcb, 'mask')
      | end
      mask Help: The PRODUCT block is used to multiply inputs.
  zECEF : Product  Tag=MBDLibrary v2007b.1  OutDataType=fixdt(1,16,0)  OutScaling=[]  RndMeth=Zero  InputSameDT=on  mask(Product (MBDLibrary)){Inputs_mbdlib=2}
      mask prompts: Inputs_mbdlib "Number of Inputs"
      mask help: Multiplies inputs.
      settings: OpenFcn=|
      | if exist('mbdlib_dialog')
      |    mbdlib_dialog(gcb,'open')
      | else
      |    open_system(gcb, 'mask')
      | end
      mask Help: The PRODUCT block is used to multiply inputs.
  geoToECEFLibOutX : Outport  OutDataType=fixdt(1,16,0)  OutScaling=[]
  geoToECEFLibOutY : Outport  Port=2  OutDataType=fixdt(1,16,0)  OutScaling=[]
  geoToECEFLibOutZ : Outport  Port=3  OutDataType=fixdt(1,16,0)  OutScaling=[]
  wires:
  Trigonometric Function3/1 -> zECEF/2, square/1(squareLibIn)
  zECEF/1 -> geoToECEFLibOutZ/1
  yECEF/1 -> geoToECEFLibOutY/1
  xECEF/1 -> geoToECEFLibOutX/1
  radius1/1 -> zECEF/1
  eqPlane/1 -> yECEF/2, xECEF/1
  Trigonometric Function2/1 -> yECEF/1
  geoToECEFLibInLon/1 -> Trigonometric Function1/1, Trigonometric Function2/1
  axisRatio/1 -> radius1/2
  geoToECEFLibInAlt/1 -> radius1/1, radius/2
  gain/1 -> axisRatio/1, radius/1
  Trigonometric Function/1 -> eqPlane/1
  Trigonometric Function1/1 -> xECEF/2
  radius/1 -> eqPlane/2
  bias/1 -> Sqrt/1
  firstEccentricitySquared/1 -> bias/1
  square/1(squareLibOut) -> firstEccentricitySquared/1
  geoToECEFLibInLat/1 -> Trigonometric Function/1, Trigonometric Function3/1
  Sqrt/1 -> Math Function/1
  Math Function/1 -> gain/1

== system SimpleEKF_2007a/INS/Attitude update/Stage1/Subsystem ==
  Quat : Inport  PortDimensions=4  OutDataType=fixdt(1,16,0)  OutScaling=[]
  Subsystem : Subsystem
  a11 : Subsystem  InitFcn=%hwbcalib_subsystem(gcbh,99);
      settings: AttributesFormatString=(Page 13)  CopyFcn=hwbcalib_copyfcn(gcbh);  DeleteFcn=hwbcalib_subsystem(gcbh,'delete');
      mask Type: Subsystem (HW)
      mask Display:
      | port_label('input',1,'quat');
      | port_label('output',1,'a11');
  a12 : Subsystem  InitFcn=%hwbcalib_subsystem(gcbh,99);
      settings: AttributesFormatString=(Page 14)  CopyFcn=hwbcalib_copyfcn(gcbh);  DeleteFcn=hwbcalib_subsystem(gcbh,'delete');
      mask Type: Subsystem (HW)
      mask Display:
      | port_label('input',1,'quat');
      | port_label('output',1,'a12');
  a13 : Subsystem  InitFcn=%hwbcalib_subsystem(gcbh,99);
      settings: AttributesFormatString=(Page 15)  CopyFcn=hwbcalib_copyfcn(gcbh);  DeleteFcn=hwbcalib_subsystem(gcbh,'delete');
      mask Type: Subsystem (HW)
      mask Display:
      | port_label('input',1,'quat');
      | port_label('output',1,'a13');
  a21 : Subsystem  InitFcn=%hwbcalib_subsystem(gcbh,99);
      settings: AttributesFormatString=(Page 16)  CopyFcn=hwbcalib_copyfcn(gcbh);  DeleteFcn=hwbcalib_subsystem(gcbh,'delete');
      mask Type: Subsystem (HW)
      mask Display:
      | port_label('input',1,'quat');
      | port_label('output',1,'a21');
  a22 : Subsystem  InitFcn=%hwbcalib_subsystem(gcbh,99);
      settings: AttributesFormatString=(Page 17)  CopyFcn=hwbcalib_copyfcn(gcbh);  DeleteFcn=hwbcalib_subsystem(gcbh,'delete');
      mask Type: Subsystem (HW)
      mask Display:
      | port_label('input',1,'quat');
      | port_label('output',1,'a22');
  a23 : Subsystem  InitFcn=%hwbcalib_subsystem(gcbh,99);
      settings: AttributesFormatString=(Page 18)  CopyFcn=hwbcalib_copyfcn(gcbh);  DeleteFcn=hwbcalib_subsystem(gcbh,'delete');
      mask Type: Subsystem (HW)
      mask Display:
      | port_label('input',1,'quat');
      | port_label('output',1,'a23');
  a31 : Subsystem  InitFcn=%hwbcalib_subsystem(gcbh,99);
      settings: AttributesFormatString=(Page 19)  CopyFcn=hwbcalib_copyfcn(gcbh);  DeleteFcn=hwbcalib_subsystem(gcbh,'delete');
      mask Type: Subsystem (HW)
      mask Display:
      | port_label('input',1,'quat');
      | port_label('output',1,'a31');
  a32 : Subsystem  InitFcn=%hwbcalib_subsystem(gcbh,99);
      settings: AttributesFormatString=(Page 20)  CopyFcn=hwbcalib_copyfcn(gcbh);  DeleteFcn=hwbcalib_subsystem(gcbh,'delete');
      mask Type: Subsystem (HW)
      mask Display:
      | port_label('input',1,'quat');
      | port_label('output',1,'a32');
  a33 : Subsystem  InitFcn=%hwbcalib_subsystem(gcbh,99);
      settings: AttributesFormatString=(Page 21)  CopyFcn=hwbcalib_copyfcn(gcbh);  DeleteFcn=hwbcalib_subsystem(gcbh,'delete');
      mask Type: Subsystem (HW)
      mask Display:
      | port_label('input',1,'quat');
      | port_label('output',1,'a33');
  quat normalize : Subsystem
  DCM : Outport  PortDimensions=[3,3]  OutDataType=fixdt(1,16,0)  OutScaling=[]  InitialOutput=0
  wires:
  Quat/1 -> quat normalize/1(q)
  Subsystem/1(Matrix) -> DCM/1
  quat normalize/1(normal(q)) -> a11/1(quat), a21/1(quat), a31/1(quat), a12/1(quat), a22/1(quat), a32/1(quat), a13/1(quat), a23/1(quat), a33/1(quat)
  a11/1(a11) -> Subsystem/1(M11)
  a21/1(a21) -> Subsystem/2(M21)
  a31/1(a31) -> Subsystem/3(M31)
  a12/1(a12) -> Subsystem/4(M12)
  a22/1(a22) -> Subsystem/5(M22)
  a32/1(a32) -> Subsystem/6(M32)
  a13/1(a13) -> Subsystem/7(M13)
  a23/1(a23) -> Subsystem/8(M23)
  a33/1(a33) -> Subsystem/9(M33)

== system SimpleEKF_2007a/INS/Attitude update/Stage1/Subsystem1 ==
  attInitCon : Inport  OutDataType=fixdt(1,16,0)  OutScaling=[]
  Mux : Mux
  a1 : Subsystem
  a2 : Subsystem
  a3 : Subsystem
  a4 : Subsystem
  q : Outport  OutDataType=fixdt(1,16,0)  OutScaling=[]
  wires:
  a1/1(a1) -> Mux/1
  a2/1(a2) -> Mux/2
  a3/1(a3) -> Mux/3
  a4/1(a2) -> Mux/4
  Mux/1 -> q/1
  attInitCon/1 -> a1/1(attInitCon), a3/1(attInitCon), a4/1(attInitCon), a2/1(attInitCon)
